simulink model "induction_Motor_Torque_stepped"  (Simulink 7.6)
settings: Solver=ode23tb  SolverMode=SingleTasking  StartTime=0.0  StopTime=3  MaxStep=10e-6  RelTol=1e-4
libraries: powerlib x9
Description:
  | Copyright 2008-2010 The MathWorks, Inc.
settings Model: Creator=MathWorks  LastModifiedBy=kif  ExtModeTrigMode=oneshot  ExtModeArmWhenConnect=off  ExtModeAutoUpdateStatusClock=off
settings DataIOCC: ExternalInput=[]  LimitDataPoints=off  SaveOutput=off  TimeSaveName=t  SignalLoggingName=sigsOut
settings OptimizationCC: BlockReduction=off  BooleanDataType=off  InlineInvariantSignals=on  InitFltsAndDblsToZero=on  EfficientMapNaN2IntZero=off
settings DebuggingCC: CheckExecutionContextPreStartOutputMsg=on  CheckExecutionContextRuntimeOutputMsg=on  SignalResolutionControl=TryResolveAllWithWarning  SolverPrmCheckMsg=none  MultiTaskDSMMsg=warning  MultiTaskCondExecSysMsg=none  SigSpecEnsureSampleTimeMsg=none  UnconnectedInputMsg=none  UnconnectedOutputMsg=none  StrictBusMsg=None
settings HardwareCC: TargetUnknown=on
settings RTWCC: IncludeERTFirstTime=on

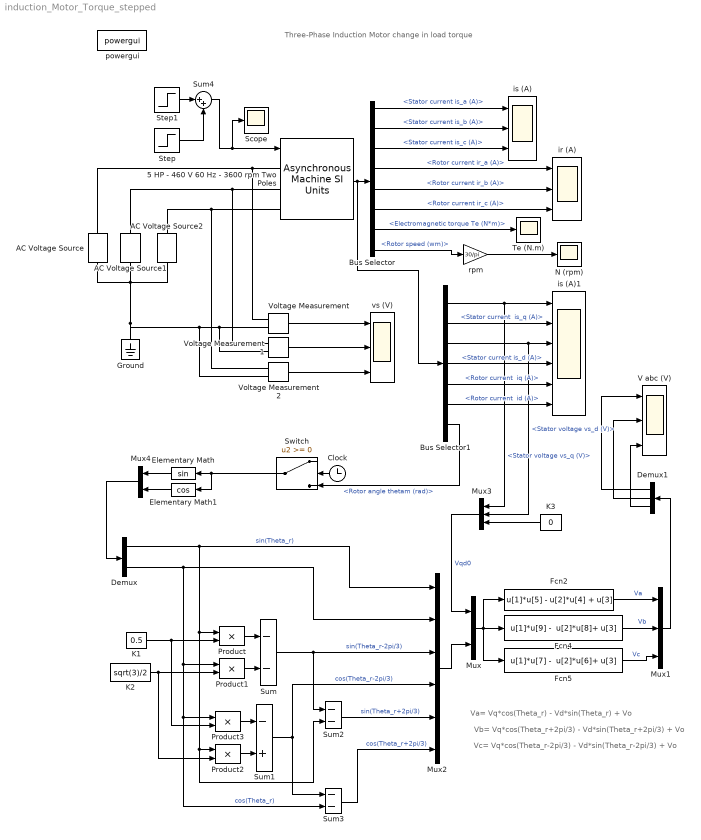
== system induction_Motor_Torque_stepped ==
  note: Three-Phase Induction Motor change in load torque
  note: Va= Vq*cos(Theta_r) - Vd*sin(Theta_r) + Vo
  note: Vc= Vq*cos(Theta_r-2pi/3) - Vd*sin(Theta_r-2pi/3) + Vo
  note: Vb= Vq*cos(Theta_r+2pi/3) - Vd*sin(Theta_r+2pi/3) + Vo
  5 HP - 460 V 60 Hz - 3600 rpm Two Poles : powerlib/Machines/Asynchronous Machine SI Units  DialogController=POWERSYS.PowerSysDialog  SystemSampleTime=-1  PresetModel=No  MechanicalLoad=Torque Tm  ShowDetailedParameters=on  RotorType=Squirrel-cage  ReferenceFrame=Stationary  NominalParameters=[3730 460 60]  Stator=[1.115 0.005974]  Rotor=[1.083 0.005974]  Cage1=[ 0.022 0.226/377]  Cage2=[ 0.022 0.226/377]  Lm=0.2037  Mechanical=[0.02 0.005752 1]  PolePairs=1  InitialConditions="[ 1,0   0,0,0   0,0,0 ]"  Units=SI  LoadFlowParameters=0  SimulateSaturation=off  Saturation=[14.03593122, 27.81365428, 53.79336849, 72.68890987, 97.98006896, 148.6815601, 215.7428561, 302.9841135, 428.7778367 ; 230, 322, 414, 460, 506, 552, 598, 644, 690]  TsPowergui=0  TsBlock=-1  IterativeModel=Forward Euler
  AC Voltage Source : powerlib/Electrical Sources/AC Voltage Source  DialogController=POWERSYS.PowerSysDialog  SystemSampleTime=-1  Amplitude=265.5  Phase=0  Frequency=60  SampleTime=0  Measurements=None
  AC Voltage Source1 : powerlib/Electrical Sources/AC Voltage Source  DialogController=POWERSYS.PowerSysDialog  SystemSampleTime=-1  Amplitude=265.5  Phase=-120  Frequency=60  SampleTime=0  Measurements=None
  AC Voltage Source2 : powerlib/Electrical Sources/AC Voltage Source  DialogController=POWERSYS.PowerSysDialog  SystemSampleTime=-1  Amplitude=265.5  Phase=120  Frequency=60  SampleTime=0  Measurements=None
  Bus Selector : BusSelector  OutputSignals=Stator measurements.Stator current is_a (A),Stator measurements.Stator current is_b (A),Stator measurements.Stator current is_c (A),Rotor measurements.Rotor current ir_a (A),Rotor measurements.Rotor current ir_b (A),Rotor measurements.Rotor current ir_c (A),Mechanical.Electromagnetic torque Te (N*m),Mechanical.Rotor speed (wm)
  Bus Selector1 : BusSelector  OutputSignals="Stator measurements.Stator voltage vs_q (V),Stator measurements.Stator current  is_q (A),Stator measurements.Stator voltage vs_d (V),Stator measurements.Stator current is_d (A),Rotor measurements.Rotor current  iq (A),Rotor measurements.Rotor current  id (A),Mechanical.Rotor angle thetam (rad)"
  Clock : Clock
      settings: Decimation=10
  Demux : Demux  Outputs=2
  Demux1 : Demux  Outputs=3
  Elementary Math : Trigonometry
  Elementary Math1 : Trigonometry  Operator=cos
  Fcn2 : Fcn  Expr="u[1]*u[5] -  u[2]*u[4] + u[3]"
  Fcn4 : Fcn  Expr="u[1]*u[9] -  u[2]*u[8]+ u[3]"
  Fcn5 : Fcn  Expr="u[1]*u[7] -  u[2]*u[6]+ u[3]"
  Ground : powerlib/Elements/Ground  DialogController=POWERSYS.PowerSysDialog  PhysicalDomain=powersysdomain  SubClassName=unknown  LeftPortType=p1  RightPortType=p1  LConnTagsString=a
  K1 : Constant  Value=0.5
  K2 : Constant  Value=sqrt(3)/2
  K3 : Constant  Value=0
  Mux : Mux  Inputs=2
  Mux1 : Mux  Inputs=3
  Mux2 : Mux  Inputs=6
  Mux3 : Mux  Inputs=3
  Mux4 : Mux  Inputs=2
  N (rpm) : Scope
      settings: TimeRange=1  YMin=0  YMax=4000  DataFormat=Structure
  Product{,1..3} (4 alike) : Product  SaturateOnIntegerOverflow=on  InputSameDT=on  OutDataTypeStr=Inherit: Same as first input
  Scope : Scope
      settings: SaveName=ScopeData6
  Step : Step  Before=5  After=10  SampleTime=1
  Step1 : Step  Time=2  After=-5  SampleTime=1
  Sum : Sum  Inputs=--  SaturateOnIntegerOverflow=on  InputSameDT=on  OutDataTypeStr=Inherit: Same as first input
  Sum1 : Sum  Inputs=-+  SaturateOnIntegerOverflow=on  InputSameDT=on  OutDataTypeStr=Inherit: Same as first input
  Sum2 : Sum  Inputs=--  SaturateOnIntegerOverflow=on  InputSameDT=on  OutDataTypeStr=Inherit: Same as first input
  Sum3 : Sum  Inputs=--  SaturateOnIntegerOverflow=on  InputSameDT=on  OutDataTypeStr=Inherit: Same as first input
  Sum4 : Sum  Inputs=|++
  Switch : Switch
  Te (N.m) : Scope
      settings: YMin=6  YMax=14  DataFormat=Structure
  V abc (V) : Scope  NumInputPorts=3
      settings: YMin=-3.5~-5~-5  YMax=3.5~5~5  SaveName=ScopeData5  DataFormat=Structure
  Voltage Measurement : powerlib/Measurements/Voltage Measurement  DialogController=POWERSYS.PowerSysDialog  SystemSampleTime=-1  PhasorSimulation=off  OutputType=Complex  PSBequivalent=0
  Voltage Measurement1 : powerlib/Measurements/Voltage Measurement  DialogController=POWERSYS.PowerSysDialog  SystemSampleTime=-1  PhasorSimulation=off  OutputType=Complex  PSBequivalent=0
  Voltage Measurement2 : powerlib/Measurements/Voltage Measurement  DialogController=POWERSYS.PowerSysDialog  SystemSampleTime=-1  PhasorSimulation=off  OutputType=Complex  PSBequivalent=0
  ir (A) : Scope  NumInputPorts=3
      settings: YMin=-3.5~-5~-5  YMax=3.5~5~5  SaveName=ScopeData2  DataFormat=Structure
  is (A) : Scope  NumInputPorts=3
      settings: YMin=-75~-75~-75  YMax=75~75~75  DataFormat=Structure
  is (A)1 : Scope  NumInputPorts=6
      settings: YMin=-300~-75~-300~-75~-75~-75  YMax=300~75~300~75~75~75  SaveName=ScopeData4  DataFormat=Structure
  powergui : powerlib/powergui  SystemSampleTime=-1  SimulationMode=Continuous  SampleTime=0  frequency=60  SPID=off  DisableSnubberDevices=off  DisableRonSwitches=off  DisableVfSwitches=off  SwTol=0  Interpol=off  frequencyindice=60  echomessages=off  HookPort=off  DisplayEquations=off  FunctionMessages=off  EnableUseOfTLC=off  x0status=blocks  RestoreLinks=warning  ResistiveCurrentMeasurement=off  Frange=[0:2:500]  Ylog=off  Xlog=on  ShowGrid=off  save=off  variable=ZData  ZoomFFT=on  StartTime=0.0  cycles=1  DisplayStyle=1  fundamental=60  FreqAxis=off  MaxFrequency=1000  frequencyindicesteady=1  RmsSteady=1  display=off  Ts=0  methode=off
  rpm : Gain  Gain=30/pi  SaturateOnIntegerOverflow=on  OutDataTypeStr=Inherit: Same as input  ParamDataTypeStr=Inherit: Same as input
  vs (V) : Scope  NumInputPorts=3
      settings: YMin=-3.5~-5~-5  YMax=3.5~5~5  SaveName=ScopeData3  DataFormat=Structure
  wires:
  Bus Selector/7 -> Te (N.m)/1  "<Electromagnetic torque Te (N*m)>"
  rpm/1 -> N (rpm)/1
  5 HP - 460 V 60 Hz - 3600 rpm Two Poles/1 -> Bus Selector/1, Bus Selector1/1
  Bus Selector/8 -> rpm/1  "<Rotor speed (wm)>"
  Bus Selector/1 -> is (A)/1  "<Stator current is_a (A)>"
  Bus Selector/2 -> is (A)/2  "<Stator current is_b (A)>"
  Bus Selector/3 -> is (A)/3  "<Stator current is_c (A)>"
  Bus Selector/4 -> ir (A)/1  "<Rotor current ir_a (A)>"
  Bus Selector/5 -> ir (A)/2  "<Rotor current ir_b (A)>"
  Bus Selector/6 -> ir (A)/3  "<Rotor current ir_c (A)>"
  Voltage Measurement/1 -> vs (V)/1
  Voltage Measurement1/1 -> vs (V)/2
  Sum4/1 -> 5 HP - 460 V 60 Hz - 3600 rpm Two Poles/1, Scope/1
  Voltage Measurement2/1 -> vs (V)/3
  Bus Selector1/1 -> is (A)1/1, Mux3/1  "<Stator voltage vs_q (V)>"
  Bus Selector1/2 -> is (A)1/2  "<Stator current  is_q (A)>"
  Bus Selector1/3 -> is (A)1/3, Mux3/2  "<Stator voltage vs_d (V)>"
  Bus Selector1/6 -> is (A)1/6  "<Rotor current  id (A)>"
  Bus Selector1/5 -> is (A)1/5  "<Rotor current  iq (A)>"
  Bus Selector1/4 -> is (A)1/4  "<Stator current is_d (A)>"
  Fcn5/1 -> Mux1/3  "Vc"
  Fcn2/1 -> Mux1/1  "Va"
  Mux1/1 -> Demux1/1
  Mux/1 -> Fcn2/1, Fcn4/1, Fcn5/1
  Sum1/1 -> Sum3/1, Mux2/4  "cos(Theta_r-2pi/3)"
  Sum/1 -> Sum2/1, Mux2/3  "sin(Theta_r-2pi/3)"
  K2/1 -> Product2/2, Product1/2
  K1/1 -> Product3/2, Product/2
  Sum2/1 -> Mux2/5  "sin(Theta_r+2pi/3)"
  Sum3/1 -> Mux2/6  "cos(Theta_r+2pi/3)"
  Product2/1 -> Sum1/2
  Product3/1 -> Sum1/1
  Product1/1 -> Sum/2
  Product/1 -> Sum/1
  Demux/1 -> Mux2/1, Sum2/2, Product2/1, Product/1  "sin(Theta_r)"
  Demux/2 -> Mux2/2, Product1/1, Product3/1, Sum3/2  "cos(Theta_r)"
  Mux4/1 -> Demux/1
  Mux2/1 -> Mux/2
  Mux3/1 -> Mux/1  "Vqd0"
  Fcn4/1 -> Mux1/2  "Vb"
  K3/1 -> Mux3/3
  Bus Selector1/7 -> Switch/3  "<Rotor angle thetam (rad)>"
  Elementary Math/1 -> Mux4/1
  Elementary Math1/1 -> Mux4/2
  Switch/1 -> Elementary Math1/1, Elementary Math/1
  Clock/1 -> Switch/2
  Demux1/1 -> V abc (V)/1
  Demux1/2 -> V abc (V)/2
  Demux1/3 -> V abc (V)/3
  Step1/1 -> Sum4/1
  Step/1 -> Sum4/2
  connections:
  5 HP - 460 V 60 Hz - 3600 rpm Two Poles/LConn1 -- AC Voltage Source/RConn1 -- Voltage Measurement/LConn1
  AC Voltage Source2/RConn1 -- 5 HP - 460 V 60 Hz - 3600 rpm Two Poles/LConn3 -- Voltage Measurement2/LConn1
  5 HP - 460 V 60 Hz - 3600 rpm Two Poles/LConn2 -- AC Voltage Source1/RConn1 -- Voltage Measurement1/LConn1
  Ground/LConn1 -- AC Voltage Source1/LConn1 -- AC Voltage Source2/LConn1 -- AC Voltage Source/LConn1 -- Voltage Measurement/LConn2 -- Voltage Measurement1/LConn2 -- Voltage Measurement2/LConn2
